simulink model "LC_control_harness"  (R2023b)
settings: Solver=FixedStepAuto  StartTime=0.0  StopTime=inf  FixedStep=0.00853333  RelTol=1e-4  AbsTol=1e-6
settings Model: DataDictionary=fmuGenerationDictionay.sldd  Creator=Veimar  LastModifiedBy=Veimar
settings ConfigSet: Description=|
  | Slow task configuration for protected model and FMU generation
  | Sample frequency = 117.1875 Hz
settings SolverCC: AutoScaleAbsTol=off  AlgebraicLoopSolver=TrustRegion  MaxZcPerStep=1
settings DataIOCC: ExternalInput=[]  InitialState=[]  SaveFormat=Array  SaveOutput=off  SaveTime=off  ReturnWorkspaceOutputs=off
settings OptimizationCC: BlockReduction=off  BooleanDataType=off  ReuseModelBlockBuffer=off  ExpressionDepthLimit=2147483647  InitFltsAndDblsToZero=on
settings DebuggingCC: SaveWithParameterizedLinksMsg=none  SignalResolutionControl=TryResolveAllWithWarning  MultiTaskDSMMsg=warning  MultiTaskCondExecSysMsg=none  IntegerOverflowMsg=none  FcnCallInpInsideContextMsg=warning  UnconnectedInputMsg=warning  UnconnectedOutputMsg=warning  UnconnectedLineMsg=warning  StateNameClashWarn=warning  SFUnexpectedBacktrackingDiag=warning  SFNoUnconditionalDefaultTransitionDiag=warning  SFExecutionAtInitializationDiag=none  IntegerSaturationMsg=none  UnderSpecifiedDimensionMsg=warning  ArithmeticOperatorsInVariantConditions=warning
settings HardwareCC: ProdBitPerPointer=32  ProdBitPerSizeT=32  ProdBitPerPtrDiffT=32  ProdLargestAtomicFloat=None  ProdWordSize=32  ProdHWDeviceType=Custom Processor->Custom Processor
settings ModelReferenceCC: EnableRefExpFcnMdlSchedulingChecks=on  PropagateSignalLabelsOutOfModel=off
settings SFSimCC: SimUseLocalCustomCode=off  CustomCodeUndefinedFunction=UseInterfaceOnly
settings RTWCC: Description=FMU2CS  SystemTargetFile=fmu2cs.tlc  TemplateMakefile=fmu2cs_default_tmf  RTWUseLocalCustomCode=off  DLArmComputeVersion=19.05
settings CodeAppCC: StateflowObjectComments=on
settings GRTTargetCC: TargetLangStandard=C89/C90 (ANSI)  CombineOutputUpdateFcns=off  MatFileLogging=off
settings ConfigComp: CovMetricSettings=dw  CovSaveCumulativeToWorkspaceVar=on  CovSaveSingleToWorkspaceVar=on  CovExternalEMLEnable=off  CovSFcnEnable=off

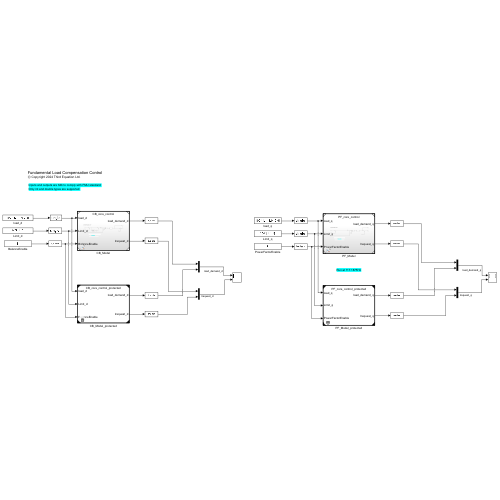
[thumbnail: Simulink's stored preview of the top-level diagram]
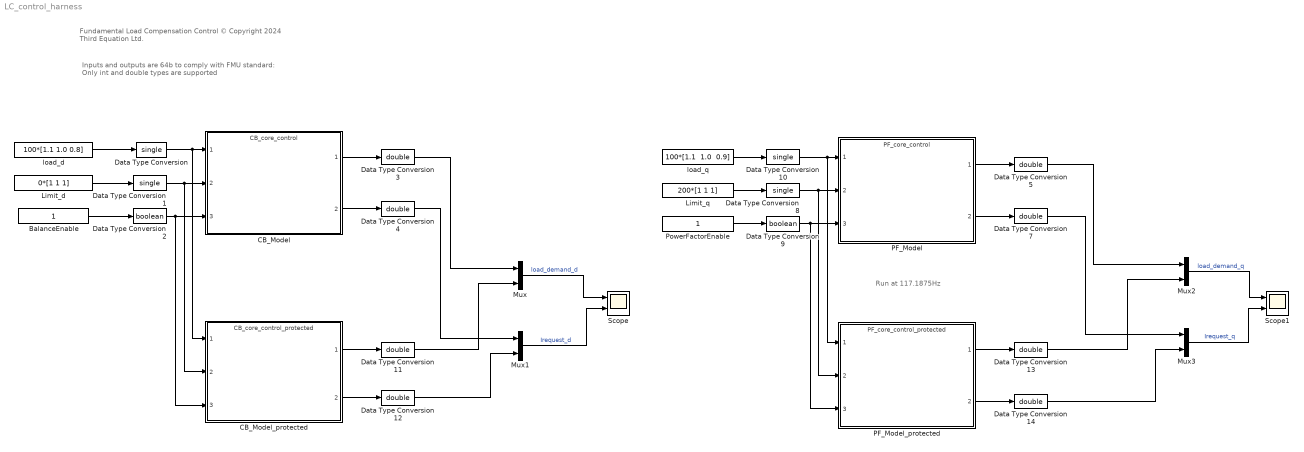
== system LC_control_harness ==
  note: Fundamental Load Compensation Control
      | © Copyright 2024 Third Equation Ltd.
  note: Inputs and outputs are 64b to comply with FMU standard:
      | Only int and double types are supported
  note: Run at 117.1875Hz
  BalanceEnable : Constant  OutDataTypeStr=int64
  CB_Model : ModelReference  ModelNameDialog=CB_core_control.slx  SimulationMode=Normal  ModelReferenceVersion=1.42
  CB_Model_protected : ModelReference  ModelNameDialog=CB_core_control_protected.slxp  ModelReferenceVersion=1.42  CopyOfModelProtected=on
  Data Type Conversion{,1,8,10} (4 alike) : DataTypeConversion  OutDataTypeStr=single  SaturateOnIntegerOverflow=off  RndMeth=Floor
  Data Type Conversion{3..5,7,11..14} (8 alike) : DataTypeConversion  OutDataTypeStr=double  SaturateOnIntegerOverflow=off  RndMeth=Floor
  Data Type Conversion2 : DataTypeConversion  OutDataTypeStr=boolean  SaturateOnIntegerOverflow=off  RndMeth=Floor
  Data Type Conversion9 : DataTypeConversion  OutDataTypeStr=boolean  SaturateOnIntegerOverflow=off  RndMeth=Floor
  Limit_d : Constant  Value=0*[1 1 1]  OutDataTypeStr=double
  Limit_q : Constant  Value=200*[1 1 1]  OutDataTypeStr=Inherit: Inherit via back propagation
  Mux{,1..3} (4 alike) : Mux  Inputs=2
  PF_Model : ModelReference  ModelNameDialog=PF_core_control.slx  SimulationMode=Normal  ModelReferenceVersion=1.42
  PF_Model_protected : ModelReference  ModelNameDialog=PF_core_control_protected.slxp  ModelReferenceVersion=1.42  CopyOfModelProtected=on
  PowerFactorEnable : Constant  OutDataTypeStr=Inherit: Inherit via back propagation
  Scope : Scope  NumInputPorts=2
  Scope1 : Scope  NumInputPorts=2
  load_d : Constant  Value=100*[1.1 1.0 0.8]  OutDataTypeStr=double
  load_q : Constant  Value="100*[1.1  1.0  0.9]"  OutDataTypeStr=Inherit: Inherit via back propagation
  wires:
  load_d/1 -> Data Type Conversion/1
  Data Type Conversion/1 -> CB_Model_protected/1, CB_Model/1
  Limit_d/1 -> Data Type Conversion1/1
  Data Type Conversion1/1 -> CB_Model_protected/2, CB_Model/2
  BalanceEnable/1 -> Data Type Conversion2/1
  Data Type Conversion2/1 -> CB_Model_protected/3, CB_Model/3
  CB_Model/1 -> Data Type Conversion3/1
  CB_Model/2 -> Data Type Conversion4/1
  Data Type Conversion4/1 -> Mux1/1
  PF_Model/2 -> Data Type Conversion7/1
  PF_Model/1 -> Data Type Conversion5/1
  Limit_q/1 -> Data Type Conversion8/1
  Data Type Conversion8/1 -> PF_Model_protected/2, PF_Model/2
  Data Type Conversion10/1 -> PF_Model_protected/1, PF_Model/1
  Data Type Conversion9/1 -> PF_Model_protected/3, PF_Model/3
  PowerFactorEnable/1 -> Data Type Conversion9/1
  load_q/1 -> Data Type Conversion10/1
  Data Type Conversion12/1 -> Mux1/2
  Data Type Conversion11/1 -> Mux/2
  CB_Model_protected/2 -> Data Type Conversion12/1
  CB_Model_protected/1 -> Data Type Conversion11/1
  PF_Model_protected/1 -> Data Type Conversion13/1
  PF_Model_protected/2 -> Data Type Conversion14/1
  Data Type Conversion13/1 -> Mux2/2
  Data Type Conversion14/1 -> Mux3/2
  Mux/1 -> Scope/1  "load_demand_d"
  Mux1/1 -> Scope/2  "Irequest_d"
  Data Type Conversion3/1 -> Mux/1
  Mux2/1 -> Scope1/1  "load_demand_q"
  Mux3/1 -> Scope1/2  "Irequest_q"
  Data Type Conversion5/1 -> Mux2/1
  Data Type Conversion7/1 -> Mux3/1
